simulink model "lung_mech_extended_variable_parameters"  (R2022b)
settings: Solver=odeN  StartTime=0.0  StopTime=10.0  MaxStep=0.01  RelTol=1e-3
model workspace: external: MATLAB File C:\Users\bigba\Dropbox\Uni\MSSF\notes\class notes\Lezione02\lung_mech_extend_parameters.m (data not in the file)
undefined symbols (not defined in the file or in its folder): out
settings Model: Creator=bigba  LastModifiedBy=zhiweigong
settings DebuggingCC: AlgebraicLoopMsg=none  UnconnectedInputMsg=warning  UnconnectedOutputMsg=warning  UnconnectedLineMsg=warning
settings ModelReferenceCC: EnableRefExpFcnMdlSchedulingChecks=on
settings RTWCC: DLArmComputeVersion=19.05

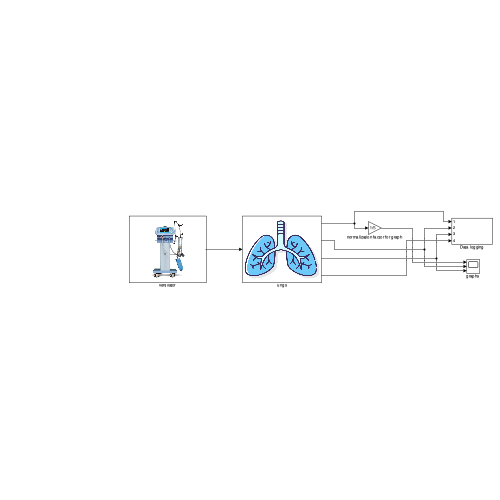
[thumbnail: Simulink's stored preview of the top-level diagram]
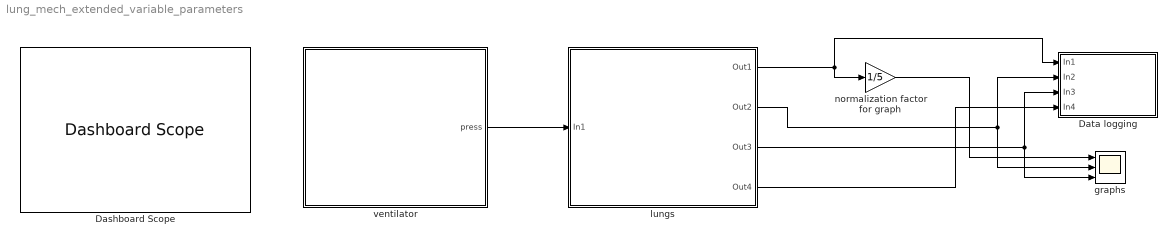
== system lung_mech_extended_variable_parameters ==
  Dashboard Scope : DashboardScope  Ymin=-10  Ymax=10  LegendPosition=Hide
  Data logging : Subsystem
  graphs : Scope  NumInputPorts=3
  lungs : Subsystem  mask{Rc=0.1, Rp=0.1, Cs=0.001, Cw=0.02, CL=0.02}
      mask prompts: Rc "Rc [cmH2O s/ L]"; Rp "Rp  [cmH2O s/ L]"; Cs "Cs [L /cmH2O ]"; Cw "Cw [L /cmH2O ]"; CL "CL [L /cmH2O ]"
      mask init:
      | STR=strcat('Rc_',num2str(Rc),'_Rp_',num2str(Rp),'_Cs_',num2str(Cs),'_Cw_',num2str(Cw),'_CL_',num2str(CL));
      | STR=strcat('data_log/data_',STR,'.mat');
      | 
      | set_param('lung_mech_extended_variable_parameters/Data logging/To File','Filename',STR)
      mask DialogControl Control2 Prompt: Reset to deafult parameters
      mask DialogControl Control2 Callback:
      | p = Simulink.Mask.get('lung_mech_extended_variable_parameters/lungs');
      | p.Parameters(1).set('Value','1'); %Rc=1;% [cmH2O s/L ] %% upper airways resistance
      | p.Parameters(2).set('Value','0.5');  % Rp=0.5; % [cmH2O s/L ] %% deeper airways resistance
      | p.Parameters(3).set('Value','0.005');  %Cs=0.005; % [ L/cmH2O ] %% shunt capacitance
      | p.Parameters(4).set('Value','0.02');  % correction SEE REPORT %CL=0.2; % [ L/cmH2O ] %% lungs capacitance
      | p.Parameters(5).set('Value','0.02');   % correction SEE REPORT   %Cw=0.2; % [ L/cmH2O ] %% pleural wall capacitance
      mask Display: image('$imagefile'); % Use "Edit Image" on toolstrip to change.
  normalization factor for graph : Gain  Gain=1/5
  ventilator : Subsystem  mask{breath_for_minute=12, flag_ventilation=3, T_insp=16.67, tau_int=15, PEEP=3, Paw=25}
      mask prompts: T_insp "Inspiratory time (% of period T)"; tau_int "Rise time (% of the inspiratory Time)"; PEEP "PEEP [cm H2O]"; Paw "PaO [cm H2O]"
      mask TypeOptions flag_ventilation: 1 | 2 | 3
      mask DialogControl Container2 Prompt: Frequency selector
      mask DialogControl Control4 Prompt: Standard: 18 breath/min
      mask DialogControl Control3 Prompt: Set respiratory frequency (breath for minute)
      mask DialogControl Container1 Prompt: Wave type
      mask DialogControl Control2 Prompt: Set:
      mask DialogControl Control7 Prompt: 1 for sine wave;
      mask DialogControl Control5 Prompt: 2 for square wave;
      mask DialogControl Control6 Prompt: 3 for square wave with rise time
      mask DialogControl Container3 Prompt: General parameters
      mask DialogControl Container6 Prompt: Time control
      mask DialogControl Container4 Prompt: Pressure control
      mask Display: image('$imagefile'); % Use "Edit Image" on toolstrip to change.
  wires:
  normalization factor for graph/1 -> graphs/1
  lungs/1(Out1) -> normalization factor for graph/1, Data logging/1(In1)
  lungs/2(Out2) -> graphs/2, Data logging/2(In2)
  lungs/3(Out3) -> graphs/3, Data logging/3(In3)
  ventilator/1(press) -> lungs/1(In1)
  lungs/4(Out4) -> Data logging/4(In4)

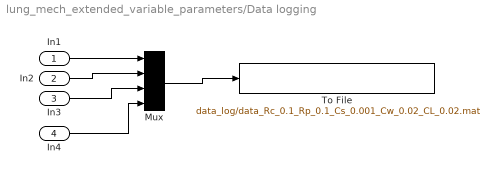
== system lung_mech_extended_variable_parameters/Data logging ==
  In1 : Inport
  In2 : Inport  Port=2
  In3 : Inport  Port=3
  In4 : Inport  Port=4
  Mux : Mux
  To File : ToFile  LoadFcn=set_param(gcb,'Filename',out.name_output);  Filename=data_log/data_Rc_0.1_Rp_0.1_Cs_0.001_Cw_0.02_CL_0.02.mat  MatrixName=mechanics_lung  SaveFormat=Timeseries
  wires:
  Mux/1 -> To File/1
  In3/1 -> Mux/3
  In2/1 -> Mux/2
  In1/1 -> Mux/1
  In4/1 -> Mux/4

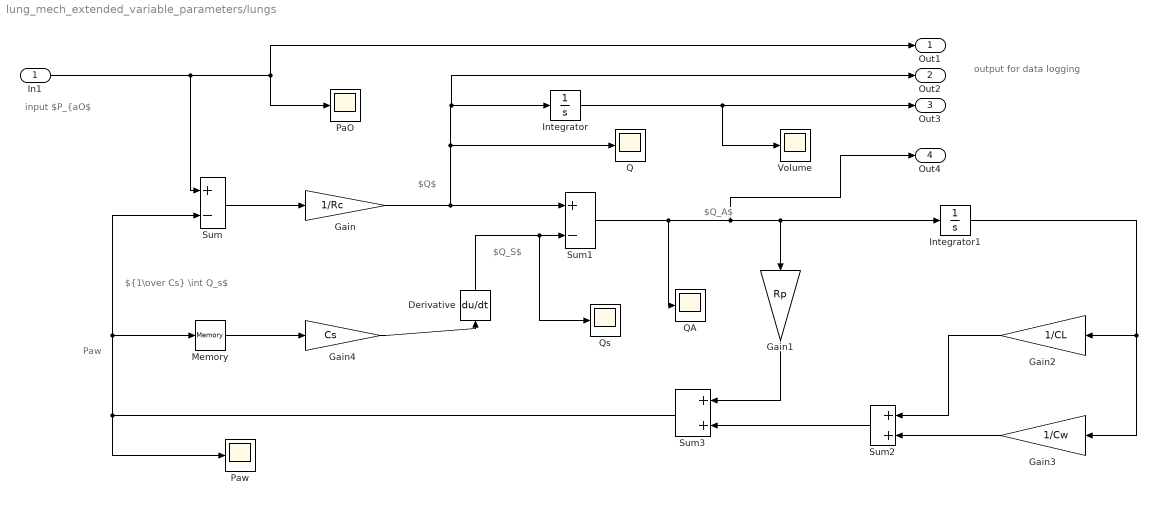
== system lung_mech_extended_variable_parameters/lungs ==
  note: output for
      | data logging
  note: input
      | $P_{aO$
  note: $Q_A$
  note: ${1\over Cs} \int Q_s$
  note: Paw
  note: $Q_S$
  note: $Q$
  In1 : Inport
  Derivative : Derivative
  Gain : Gain  Gain=1/Rc
  Gain1 : Gain  Gain=Rp
  Gain2 : Gain  Gain=1/CL
  Gain3 : Gain  Gain=1/Cw
  Gain4 : Gain  Gain=Cs
  Integrator : Integrator
  Integrator1 : Integrator
  Memory : Memory
  PaO : Scope
  Paw : Scope
  Q : Scope
  QA : Scope
  Qs : Scope
  Sum : Sum  Inputs=+-
  Sum1 : Sum  Inputs=+-
  Sum2 : Sum
  Sum3 : Sum
  Volume : Scope
  Out1 : Outport
  Out2 : Outport  Port=2
  Out3 : Outport  Port=3
  Out4 : Outport  Port=4
  wires:
  Memory/1 -> Gain4/1
  Sum3/1 -> Sum/2, Memory/1, Paw/1
  Gain/1 -> Integrator/1, Out2/1, Q/1, Sum1/1
  Gain1/1 -> Sum3/1
  Sum2/1 -> Sum3/2
  Gain3/1 -> Sum2/2
  Gain2/1 -> Sum2/1
  Integrator1/1 -> Gain3/1, Gain2/1
  Gain4/1 -> Derivative/1
  Integrator/1 -> Volume/1, Out3/1
  Sum/1 -> Gain/1
  Sum1/1 -> QA/1, Out4/1, Integrator1/1, Gain1/1
  In1/1 -> Sum/1, Out1/1, PaO/1
  Derivative/1 -> Qs/1, Sum1/2

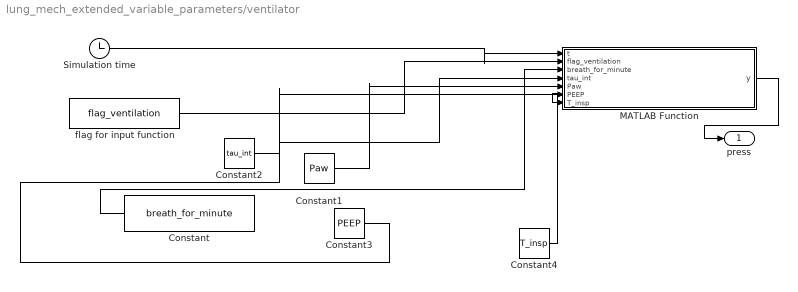
== system lung_mech_extended_variable_parameters/ventilator ==
  Constant : Constant  Value=breath_for_minute
  Constant1 : Constant  Value=Paw
  Constant2 : Constant  Value=tau_int
  Constant3 : Constant  Value=PEEP
  Constant4 : Constant  Value=T_insp
  MATLAB Function : MATLAB Function  TreatAsAtomicUnit=on
  Simulation time : Clock
  flag for input function : Constant  Value=flag_ventilation
  press : Outport
  wires:
  Simulation time/1 -> MATLAB Function/1(t)
  MATLAB Function/1(y) -> press/1
  flag for input function/1 -> MATLAB Function/2(flag_ventilation)
  Constant/1 -> MATLAB Function/3(breath_for_minute)
  Constant2/1 -> MATLAB Function/4(tau_int)
  Constant1/1 -> MATLAB Function/5(Paw)
  Constant3/1 -> MATLAB Function/6(PEEP)
  Constant4/1 -> MATLAB Function/7(T_insp)

== matlab function lung_mech_extended_variable_parameters/ventilator/MATLAB Function ==
  data: t input; y output; flag_ventilation input; breath_for_minute input; tau_int input; Paw input; PEEP input; T_insp input
function y = fcn(t,flag_ventilation,breath_for_minute,tau_int,Paw,PEEP,T_insp)

% % % to avoid error use the `odeN` solver !

f=breath_for_minute/60; % breathing frequence in Hz
% pressure diffrence from maximus value and PEEP
DeltaPressure=Paw-PEEP; 

A=0; % initialize output variable

if flag_ventilation==1 % flag=1 for sine wave
    % sine wave from Khoo Physiological Control Sistem
    % amplitude peak-peak of 5 cmH2O
    amplitude=5;
    A=amplitude*sin(2*pi*f*t);  
end

if flag_ventilation==2 % flag=2 for perfect square wave
    dt=rem(t,(1/f)); % current time (of single period)
    period=1/f; 
    half_period=period/2; % duty cycle of 50 % by selecting half period
    if  dt<half_period % semi-period where the output is on
        amplitude=5;   % amplitude of 5 [cmH2O] 
        A=amplitude; % set the output constant
    end
    if dt>= half_period % semi-period where the output is zero
        A=0; % set the output to zero 
    end 
end

if flag_ventilation==3 % flag=3 for square wave with rise time tau
    period=1/f; 
    dt=rem(t,(1/f));  % current time (of single period)
    % the inspiratory time (where the output is on) is defined 
    % usign percentage of total period with T_insp from ventilator GUI
    % also the rise time is defined using percentage of inspiratory time
    % with tau_int from ventilator GUI
    insp_Time=(T_insp/100)*period; 
    tau=(tau_int/100)*insp_Time;
    if dt < tau % rise time
        % linear growth of the pressur with offset 
        A=DeltaPressure*(dt/tau)+PEEP; 
    end
    if  (dt>=tau) && (dt<insp_Time) % the pressure is max (square wave on)
        A=DeltaPressure+PEEP;
    end
    if dt>= insp_Time %the pressure is min (square wave off)
    A=PEEP;
    end 
end

y=A; % set the pressure wave as function output

end
